simulink model "newstatefeedback"  (Simulink 5.0)
settings: Solver=ode45  StartTime=0.0  StopTime=10.0  RelTol=1e-3
InitFcn:
  | init_c
undefined symbols (not defined in the file): a, dzcv, fc, fp, fs, g, j, l, mi, xc, yc
settings Model: LastModifiedBy=AD

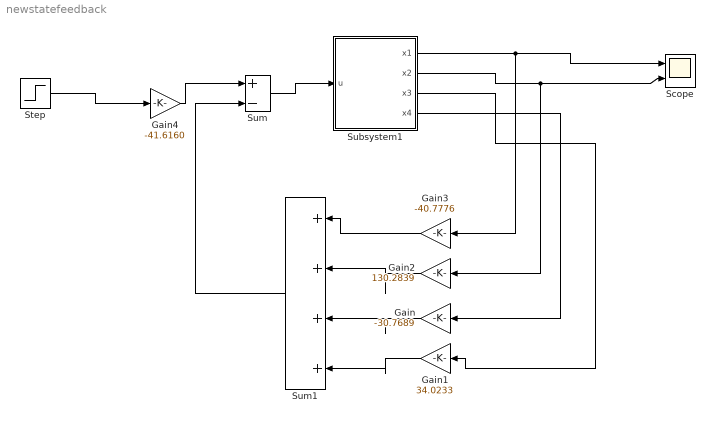
== system newstatefeedback ==
  Gain : Gain  Orientation=left  Gain=-30.7689  SaturateOnIntegerOverflow=on
  Gain1 : Gain  Orientation=left  Gain=34.0233  SaturateOnIntegerOverflow=on
  Gain2 : Gain  Orientation=left  Gain=130.2839  SaturateOnIntegerOverflow=on
  Gain3 : Gain  Orientation=left  Gain=-40.7776  SaturateOnIntegerOverflow=on
  Gain4 : Gain  Gain=-41.6160  SaturateOnIntegerOverflow=on
  Scope : Scope  NumInputPorts=2
      settings: TimeRange=10  YMin=-100~0  YMax=500~120
  Step : Step  SampleTime=0
  Subsystem1 : Subsystem
  Sum : Sum  Inputs=|+-  SaturateOnIntegerOverflow=on
  Sum1 : Sum  Orientation=left  Inputs=|++++  SaturateOnIntegerOverflow=on
  wires:
  Gain3/1 -> Sum1/1
  Gain2/1 -> Sum1/2
  Gain/1 -> Sum1/3
  Gain1/1 -> Sum1/4
  Sum1/1 -> Sum/2
  Gain4/1 -> Sum/1
  Step/1 -> Gain4/1
  Subsystem1/1(x1) -> Gain3/1, Scope/1
  Subsystem1/2(x2) -> Scope/2, Gain2/1
  Subsystem1/3(x3) -> Gain/1
  Subsystem1/4(x4) -> Gain1/1
  Sum/1 -> Subsystem1/1(u)

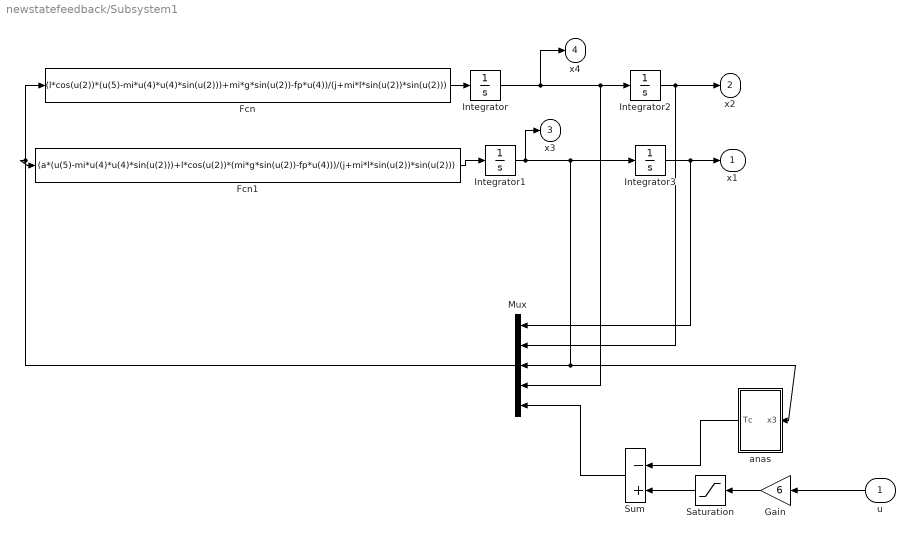
== system newstatefeedback/Subsystem1 ==
  u : Inport  Orientation=left
  Fcn : Fcn  Expr=(l*cos(u(2))*(u(5)-mi*u(4)*u(4)*sin(u(2)))+mi*g*sin(u(2))-fp*u(4))/(j+mi*l*sin(u(2))*sin(u(2)))
  Fcn1 : Fcn  Expr=(a*(u(5)-mi*u(4)*u(4)*sin(u(2)))+l*cos(u(2))*(mi*g*sin(u(2))-fp*u(4)))/(j+mi*l*sin(u(2))*sin(u(2)))
  Gain : Gain  Orientation=left  Gain=6  SaturateOnIntegerOverflow=on
  Integrator{,1..3} (4 alike) : Integrator
  Mux : Mux  Orientation=left  Inputs=5
  Saturation : Saturate  Orientation=left  UpperLimit=17  LowerLimit=-17
  Sum : Sum  Orientation=left  Inputs=|-+  SaturateOnIntegerOverflow=on
  anas : Subsystem  Orientation=left
  x1 : Outport
  x2 : Outport  Port=2
  x3 : Outport  Port=3
  x4 : Outport  Port=4
  wires:
  Fcn/1 -> Integrator/1
  Fcn1/1 -> Integrator1/1
  Integrator/1 -> Integrator2/1, Mux/4, x4/1
  Integrator1/1 -> Integrator3/1, Mux/3, anas/1(x3), x3/1
  Integrator2/1 -> x2/1, Mux/2
  Integrator3/1 -> x1/1, Mux/1
  Mux/1 -> Fcn1/1, Fcn/1
  Sum/1 -> Mux/5
  Gain/1 -> Saturation/1
  Saturation/1 -> Sum/2
  u/1 -> Gain/1
  anas/1(Tc) -> Sum/1

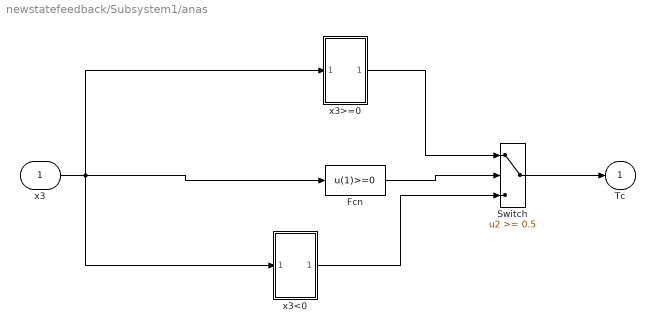
== system newstatefeedback/Subsystem1/anas ==
  x3 : Inport
  Fcn : Fcn  Expr=u(1)>=0
  Switch : Switch  Threshold=0.5  SaturateOnIntegerOverflow=on
  x3<0 : Subsystem
  x3>=0 : Subsystem
  Tc : Outport
  wires:
  Switch/1 -> Tc/1
  Fcn/1 -> Switch/2
  x3/1 -> Fcn/1, x3>=0/1(In1), x3<0/1(In1)
  x3>=0/1(out1) -> Switch/1
  x3<0/1(out1) -> Switch/3

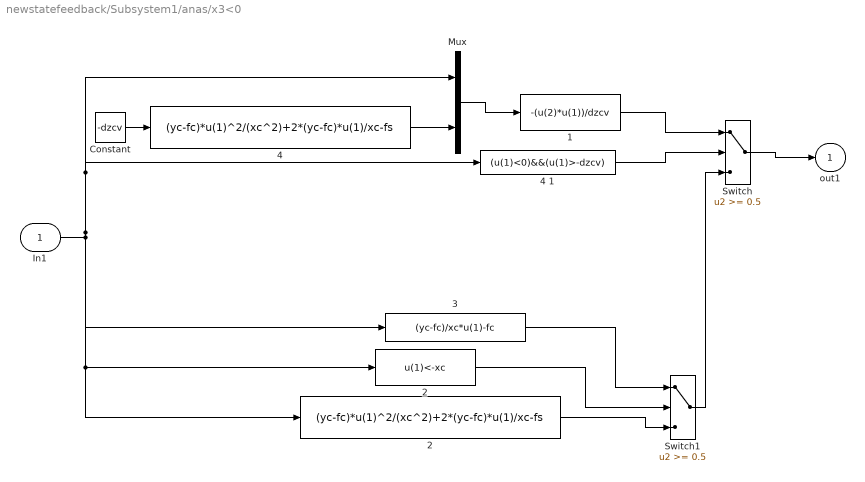
== system newstatefeedback/Subsystem1/anas/x3<0 ==
  In1 : Inport
  1 : Fcn  Expr=-(u(2)*u(1))/dzcv
  2 : Fcn  Expr=u(1)<-xc
  "2 " : Fcn  Expr=(yc-fc)*u(1)^2/(xc^2)+2*(yc-fc)*u(1)/xc-fs
  3 : Fcn  Expr=(yc-fc)/xc*u(1)-fc
  "4 " : Fcn  Expr=(yc-fc)*u(1)^2/(xc^2)+2*(yc-fc)*u(1)/xc-fs
  4 1 : Fcn  Expr=(u(1)<0)&&(u(1)>-dzcv)
  Constant : Constant  Value=-dzcv
  Mux : Mux  Inputs=2
  Switch : Switch  Threshold=0.5  SaturateOnIntegerOverflow=on
  Switch1 : Switch  Threshold=0.5  SaturateOnIntegerOverflow=on
  out1 : Outport
  wires:
  1/1 -> Switch/1
  3/1 -> Switch1/1
  2/1 -> Switch1/2
  "2 "/1 -> Switch1/3
  Switch1/1 -> Switch/3
  Mux/1 -> 1/1
  "4 "/1 -> Mux/2
  In1/1 -> 3/1, 2/1, "2 "/1, Mux/1, 4 1/1
  Constant/1 -> "4 "/1
  4 1/1 -> Switch/2
  Switch/1 -> out1/1

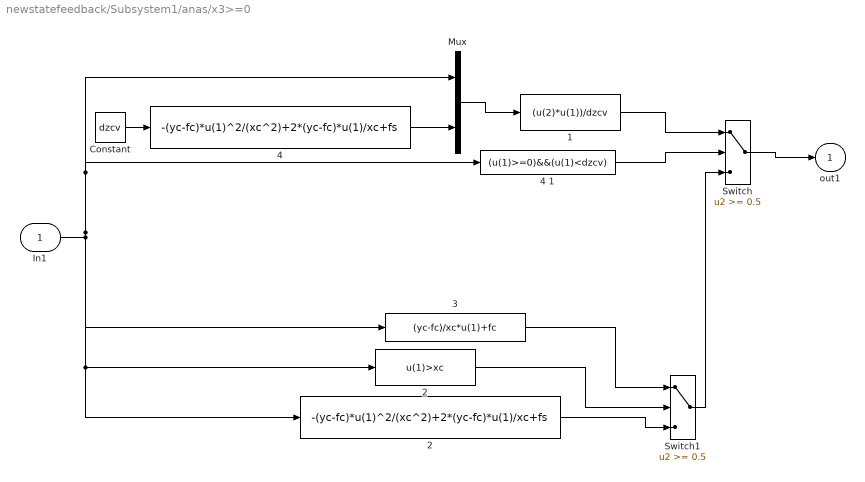
== system newstatefeedback/Subsystem1/anas/x3>=0 ==
  In1 : Inport
  1 : Fcn  Expr=(u(2)*u(1))/dzcv
  2 : Fcn  Expr=u(1)>xc
  "2 " : Fcn  Expr=-(yc-fc)*u(1)^2/(xc^2)+2*(yc-fc)*u(1)/xc+fs
  3 : Fcn  Expr=(yc-fc)/xc*u(1)+fc
  "4 " : Fcn  Expr=-(yc-fc)*u(1)^2/(xc^2)+2*(yc-fc)*u(1)/xc+fs
  4 1 : Fcn  Expr=(u(1)>=0)&&(u(1)<dzcv)
  Constant : Constant  Value=dzcv
  Mux : Mux  Inputs=2
  Switch : Switch  Threshold=0.5  SaturateOnIntegerOverflow=on
  Switch1 : Switch  Threshold=0.5  SaturateOnIntegerOverflow=on
  out1 : Outport
  wires:
  1/1 -> Switch/1
  3/1 -> Switch1/1
  2/1 -> Switch1/2
  "2 "/1 -> Switch1/3
  Switch1/1 -> Switch/3
  Mux/1 -> 1/1
  "4 "/1 -> Mux/2
  In1/1 -> 3/1, 2/1, "2 "/1, Mux/1, 4 1/1
  Constant/1 -> "4 "/1
  4 1/1 -> Switch/2
  Switch/1 -> out1/1
